simulink model "simplified_powertrain"  (R2020b)
settings: Solver=FixedStepAuto  StartTime=0.0  StopTime=60  RelTol=1e-3
PreLoadFcn:
  | C_sc = 1;
StartFcn:
  | C_sc = 1;
values from neighbouring files (symbols this model uses):
  D = 0    [model_fc.m]
undefined symbols (not defined in the file or in its folder): command, DiscIntNeverNeededParam, ECMS, Flight, in, Ion, Lithium, out, w
libraries: powerlib x22, electricdrivelib x3, lib_converters x3, simulink x2, fuzblock x1, mpclib x1, re_lib x1
(part 5 of 6)

== system simplified_powertrain/EMS/Management Variant/SMC/Discrete PI Controller1 ==
  note: Pierre Giroux, Gilbert Sybille
      | Power System Simulation Laboratory
      | IREQ, Hydro-Quebc
  note: Discrete PID Controller
  Error : Inport  SampleTime=Ts
  Discrete-Time Integrator : DiscreteIntegrator  InitialCondition=Init  SampleTime=Ts  LimitOutput=on  UpperSaturationLimit=UpperLimit  LowerSaturationLimit=LowerLimit  ICPrevOutput=DiscIntNeverNeededParam  ICPrevScaledInput=DiscIntNeverNeededParam
  Kp4 : Gain  Gain=Kp  SaturateOnIntegerOverflow=on  SampleTime=Ts  OutDataTypeStr=Inherit: Same as input  ParamDataTypeStr=Inherit: Same as input
  Kp5 : Gain  Gain=Ki  SaturateOnIntegerOverflow=on  SampleTime=Ts  OutDataTypeStr=Inherit: Same as input  ParamDataTypeStr=Inherit: Same as input
  Saturation2 : Saturate  UpperLimit=UpperLimit  LowerLimit=LowerLimit  SampleTime=Ts
  Sum6 : Sum  InputSameDT=on  SaturateOnIntegerOverflow=on  SampleTime=Ts  OutDataTypeStr=Inherit: Same as first input
  Zero-Order Hold : ZeroOrderHold  SampleTime=Ts
  Out : Outport  SampleTime=Ts  InitialOutput=0  VectorParamsAs1DForOutWhenUnconnected=off
  wires:
  Error/1 -> Kp4/1, Kp5/1
  Sum6/1 -> Saturation2/1
  Kp5/1 -> Discrete-Time Integrator/1
  Kp4/1 -> Zero-Order Hold/1
  Discrete-Time Integrator/1 -> Sum6/2
  Saturation2/1 -> Out/1
  Zero-Order Hold/1 -> Sum6/1

== system simplified_powertrain/EMS/Management Variant/SMC/Discrete PI Controller2 ==
  note: Pierre Giroux, Gilbert Sybille
      | Power System Simulation Laboratory
      | IREQ, Hydro-Quebc
  note: Discrete PID Controller
  Error : Inport  SampleTime=Ts
  Discrete-Time Integrator : DiscreteIntegrator  InitialCondition=Init  SampleTime=Ts  LimitOutput=on  UpperSaturationLimit=UpperLimit  LowerSaturationLimit=LowerLimit  ICPrevOutput=DiscIntNeverNeededParam  ICPrevScaledInput=DiscIntNeverNeededParam
  Kp4 : Gain  Gain=Kp  SaturateOnIntegerOverflow=on  SampleTime=Ts  OutDataTypeStr=Inherit: Same as input  ParamDataTypeStr=Inherit: Same as input
  Kp5 : Gain  Gain=Ki  SaturateOnIntegerOverflow=on  SampleTime=Ts  OutDataTypeStr=Inherit: Same as input  ParamDataTypeStr=Inherit: Same as input
  Saturation2 : Saturate  UpperLimit=UpperLimit  LowerLimit=LowerLimit  SampleTime=Ts
  Sum6 : Sum  InputSameDT=on  SaturateOnIntegerOverflow=on  SampleTime=Ts  OutDataTypeStr=Inherit: Same as first input
  Zero-Order Hold : ZeroOrderHold  SampleTime=Ts
  Out : Outport  SampleTime=Ts  InitialOutput=0  VectorParamsAs1DForOutWhenUnconnected=off
  wires:
  Error/1 -> Kp4/1, Kp5/1
  Sum6/1 -> Saturation2/1
  Kp5/1 -> Discrete-Time Integrator/1
  Kp4/1 -> Zero-Order Hold/1
  Discrete-Time Integrator/1 -> Sum6/2
  Saturation2/1 -> Out/1
  Zero-Order Hold/1 -> Sum6/1

== system simplified_powertrain/EMS/Management Variant/SMC/Discrete PI Controller3 ==
  note: Discrete PID Controller
  note: Pierre Giroux, Gilbert Sybille
      | Power System Simulation Laboratory
      | IREQ, Hydro-Quebc
  Error : Inport  SampleTime=Ts
  Discrete-Time Integrator : DiscreteIntegrator  InitialCondition=Init  SampleTime=Ts  LimitOutput=on  UpperSaturationLimit=UpperLimit  LowerSaturationLimit=LowerLimit  ICPrevOutput=DiscIntNeverNeededParam  ICPrevScaledInput=DiscIntNeverNeededParam
  Kp4 : Gain  Gain=Kp  SaturateOnIntegerOverflow=on  SampleTime=Ts  OutDataTypeStr=Inherit: Same as input  ParamDataTypeStr=Inherit: Same as input
  Kp5 : Gain  Gain=Ki  SaturateOnIntegerOverflow=on  SampleTime=Ts  OutDataTypeStr=Inherit: Same as input  ParamDataTypeStr=Inherit: Same as input
  Saturation2 : Saturate  UpperLimit=UpperLimit  LowerLimit=LowerLimit  SampleTime=Ts
  Sum6 : Sum  InputSameDT=on  SaturateOnIntegerOverflow=on  SampleTime=Ts  OutDataTypeStr=Inherit: Same as first input
  Zero-Order Hold : ZeroOrderHold  SampleTime=Ts
  Out : Outport  SampleTime=Ts  InitialOutput=0  VectorParamsAs1DForOutWhenUnconnected=off
  wires:
  Zero-Order Hold/1 -> Sum6/1
  Saturation2/1 -> Out/1
  Discrete-Time Integrator/1 -> Sum6/2
  Kp4/1 -> Zero-Order Hold/1
  Kp5/1 -> Discrete-Time Integrator/1
  Sum6/1 -> Saturation2/1
  Error/1 -> Kp5/1, Kp4/1

== system simplified_powertrain/EMS/Management Variant/SMC/Discrete PI Controller5 ==
  note: Pierre Giroux, Gilbert Sybille
      | Power System Simulation Laboratory
      | IREQ, Hydro-Quebc
  note: Discrete PID Controller
  Error : Inport  SampleTime=Ts
  Discrete-Time Integrator : DiscreteIntegrator  InitialCondition=Init  SampleTime=Ts  LimitOutput=on  UpperSaturationLimit=UpperLimit  LowerSaturationLimit=LowerLimit  ICPrevOutput=DiscIntNeverNeededParam  ICPrevScaledInput=DiscIntNeverNeededParam
  Kp4 : Gain  Gain=Kp  SaturateOnIntegerOverflow=on  SampleTime=Ts  OutDataTypeStr=Inherit: Same as input  ParamDataTypeStr=Inherit: Same as input
  Kp5 : Gain  Gain=Ki  SaturateOnIntegerOverflow=on  SampleTime=Ts  OutDataTypeStr=Inherit: Same as input  ParamDataTypeStr=Inherit: Same as input
  Saturation2 : Saturate  UpperLimit=UpperLimit  LowerLimit=LowerLimit  SampleTime=Ts
  Sum6 : Sum  InputSameDT=on  SaturateOnIntegerOverflow=on  SampleTime=Ts  OutDataTypeStr=Inherit: Same as first input
  Zero-Order Hold : ZeroOrderHold  SampleTime=Ts
  Out : Outport  SampleTime=Ts  InitialOutput=0  VectorParamsAs1DForOutWhenUnconnected=off
  wires:
  Error/1 -> Kp4/1, Kp5/1
  Sum6/1 -> Saturation2/1
  Kp5/1 -> Discrete-Time Integrator/1
  Kp4/1 -> Zero-Order Hold/1
  Discrete-Time Integrator/1 -> Sum6/2
  Saturation2/1 -> Out/1
  Zero-Order Hold/1 -> Sum6/1

== system simplified_powertrain/EMS/Management Variant/SMC/Discrete PI Controller6 ==
  note: Discrete PID Controller
  note: Pierre Giroux, Gilbert Sybille
      | Power System Simulation Laboratory
      | IREQ, Hydro-Quebc
  Error : Inport  SampleTime=Ts
  Discrete-Time Integrator : DiscreteIntegrator  InitialCondition=Init  SampleTime=Ts  LimitOutput=on  UpperSaturationLimit=UpperLimit  LowerSaturationLimit=LowerLimit  ICPrevOutput=DiscIntNeverNeededParam  ICPrevScaledInput=DiscIntNeverNeededParam
  Kp4 : Gain  Gain=Kp  SaturateOnIntegerOverflow=on  SampleTime=Ts  OutDataTypeStr=Inherit: Same as input  ParamDataTypeStr=Inherit: Same as input
  Kp5 : Gain  Gain=Ki  SaturateOnIntegerOverflow=on  SampleTime=Ts  OutDataTypeStr=Inherit: Same as input  ParamDataTypeStr=Inherit: Same as input
  Saturation2 : Saturate  UpperLimit=UpperLimit  LowerLimit=LowerLimit  SampleTime=Ts
  Sum6 : Sum  InputSameDT=on  SaturateOnIntegerOverflow=on  SampleTime=Ts  OutDataTypeStr=Inherit: Same as first input
  Zero-Order Hold : ZeroOrderHold  SampleTime=Ts
  Out : Outport  SampleTime=Ts  InitialOutput=0  VectorParamsAs1DForOutWhenUnconnected=off
  wires:
  Zero-Order Hold/1 -> Sum6/1
  Saturation2/1 -> Out/1
  Discrete-Time Integrator/1 -> Sum6/2
  Kp4/1 -> Zero-Order Hold/1
  Kp5/1 -> Discrete-Time Integrator/1
  Sum6/1 -> Saturation2/1
  Error/1 -> Kp5/1, Kp4/1

== system simplified_powertrain/EMS/Management Variant/SMC/Discrete PI Controller7 ==
  note: Pierre Giroux, Gilbert Sybille
      | Power System Simulation Laboratory
      | IREQ, Hydro-Quebc
  note: Discrete PID Controller
  Error : Inport  SampleTime=Ts
  Discrete-Time Integrator : DiscreteIntegrator  InitialCondition=Init  SampleTime=Ts  LimitOutput=on  UpperSaturationLimit=UpperLimit  LowerSaturationLimit=LowerLimit  ICPrevOutput=DiscIntNeverNeededParam  ICPrevScaledInput=DiscIntNeverNeededParam
  Kp4 : Gain  Gain=Kp  SaturateOnIntegerOverflow=on  SampleTime=Ts  OutDataTypeStr=Inherit: Same as input  ParamDataTypeStr=Inherit: Same as input
  Kp5 : Gain  Gain=Ki  SaturateOnIntegerOverflow=on  SampleTime=Ts  OutDataTypeStr=Inherit: Same as input  ParamDataTypeStr=Inherit: Same as input
  Saturation2 : Saturate  UpperLimit=UpperLimit  LowerLimit=LowerLimit  SampleTime=Ts
  Sum6 : Sum  InputSameDT=on  SaturateOnIntegerOverflow=on  SampleTime=Ts  OutDataTypeStr=Inherit: Same as first input
  Zero-Order Hold : ZeroOrderHold  SampleTime=Ts
  Out : Outport  SampleTime=Ts  InitialOutput=0  VectorParamsAs1DForOutWhenUnconnected=off
  wires:
  Error/1 -> Kp4/1, Kp5/1
  Sum6/1 -> Saturation2/1
  Kp5/1 -> Discrete-Time Integrator/1
  Kp4/1 -> Zero-Order Hold/1
  Discrete-Time Integrator/1 -> Sum6/2
  Saturation2/1 -> Out/1
  Zero-Order Hold/1 -> Sum6/1

== matlab function simplified_powertrain/EMS/Management Variant/SMC/MATLAB Function ==
  settings: updateMethod=DISCRETE  sampleTime=Ts
  data: Vbatt input; Ibatt input; Ibatt_out input; Ibatt_1 output; Ifc_out input; Vpv input; Ipv input; Ipv_out input; Pload input; Vdc input; Vdc_wanted input; Pout input; Ibatt_2 output; Ibatt_3 output; IO_batt_conv output; IO_batt_conv_value input; Ifc_boost input; Vfc input
function [Ibatt_1, Ibatt_2, Ibatt_3,  IO_batt_conv] = fcn(Vbatt, Ibatt,Ibatt_out, Ifc_out, Vpv, Ipv, Ipv_out,Pload,Vdc,Vdc_wanted, Pout, IO_batt_conv_value, Ifc_boost, Vfc)
    %% Part - 1
    %     FC = Vfc * Ifc_boost;
    %     FC = Vfc * Ifc_in;
    %     FC = Vdc_wanted * Ifc_out;
    FC = Vdc * Ifc_out;
    
    %     PV = Vpv * Ipv_boost;
%         PV = Vpv * Ipv; % stable pv panel but not good
    %     PV = Vdc_wanted * Ipv_out;
    PV = Vdc * Ipv_out; % marche mieux avec celui ci mais pv pas au max
    
    %     Batt = Vbatt * Ibatt;
    Batt = Vdc * Ibatt_out;
    
    %     Ibatt_1 = (Pload - FC - PV)/Vdc_wanted;
    %     Ibatt_1 = (Pload - FC - PV)/Vdc;
    Ibatt_1 = (Pload - FC - PV - Batt)/Vdc;
    %     Ibatt_1 = -10;
    
    %% Part - 2
    Ibatt_2 = Pload - Pout;
    
    %% Part - 3
    Ibatt_3 = Vdc_wanted - Vdc;
    
    %% Activate conv
    IO_batt_conv = IO_batt_conv_value;
end

== matlab function simplified_powertrain/MATLAB Function1 ==
  data: Pfc_in input; FC output; Pfc_out input; Pbatt_in input; Pbatt_out input; Ppv_in input; Ppv_out input; BATT output; PV output
function [FC,BATT,PV] = fcn(Pfc_in,Pfc_out,Pbatt_in,Pbatt_out,Ppv_in,Ppv_out)

    FC = 100*Pfc_out/Pfc_in;
    BATT = 100*Pbatt_out/Pbatt_in;
    PV = 100*Ppv_out/Ppv_in;
    
    if FC > 100
        FC = 100;
    end
    if FC< 0
        FC = 0;
    end
    if BATT > 100
        BATT = 100;
    end
    if BATT< 0
        BATT = 0;
    end
    if PV > 100
        PV = 100;
    end
    if PV< 0
        PV = 0;
    end
    
end

== matlab function simplified_powertrain/EMS/Management Variant/FUZZY/MATLAB Function ==
  settings: updateMethod=DISCRETE  sampleTime=Ts
  data: Vbatt input; Ibatt input; Ibatt_out input; Ibatt_1 output; Ifc_out input; Vpv input; Ipv input; Ipv_out input; Pload input; Vdc input; Vdc_wanted input; Pout input; Ibatt_2 output; Ibatt_3 output; IO_batt_conv output; IO_batt_conv_value input; Ifc_boost input; Vfc input
function [Ibatt_1, Ibatt_2, Ibatt_3,  IO_batt_conv] = fcn(Vbatt, Ibatt,Ibatt_out, Ifc_out, Vpv, Ipv, Ipv_out,Pload,Vdc,Vdc_wanted, Pout, IO_batt_conv_value, Ifc_boost, Vfc)
    %% Part - 1
    %     FC = Vfc * Ifc_boost;
    %     FC = Vfc * Ifc_in;
    %     FC = Vdc_wanted * Ifc_out;
    FC = Vdc * Ifc_out;
    
    %     PV = Vpv * Ipv_boost;
%         PV = Vpv * Ipv; % stable pv panel but not good
    %     PV = Vdc_wanted * Ipv_out;
    PV = Vdc * Ipv_out; % marche mieux avec celui ci mais pv pas au max
    
    %     Batt = Vbatt * Ibatt;
    Batt = Vdc * Ibatt_out;
    
    %     Ibatt_1 = (Pload - FC - PV)/Vdc_wanted;
    %     Ibatt_1 = (Pload - FC - PV)/Vdc;
    Ibatt_1 = (Pload - FC - PV - Batt)/Vdc;
    %     Ibatt_1 = -10;
    
    %% Part - 2
    Ibatt_2 = Pload - Pout;
    
    %% Part - 3
    Ibatt_3 = Vdc_wanted - Vdc;
    
    %% Activate conv
    IO_batt_conv = IO_batt_conv_value;
end

== matlab function simplified_powertrain/EMS/Management Variant/FUZZY/MATLAB Function1 ==
  settings: updateMethod=DISCRETE  sampleTime=Ts
  data: current_comm input; conv output; Pload input; Vbus_required input; current_command output; V_batt_conv output
function [conv, current_command,V_batt_conv] = fcn(current_comm, Pload, Vbus_required)
    if current_comm < 0
        conv = 1;
        V_batt_conv = Vbus_required; % (55)
%         V_batt_conv = 55; % (55)
    else
        conv = 0;
        V_batt_conv = Vbus_required;
    end
%     V_batt_conv = 120;
    current_command = current_comm;
end

%     if Pload == 0 || current_comm < 0
%         conv = 1;
%         V_batt_conv = 50;
%     else
%         conv = 0;
%         V_batt_conv = Vbus_required;
%     end
%     current_command = current_comm;

== matlab function simplified_powertrain/EMS/Management Variant/FUZZY/PV - FC - control ==
  settings: updateMethod=DISCRETE  sampleTime=Ts
  data: Time input; Vdc_command input; Vfc input; Ifc_in input; Vbatt input; Ibatt_in input; Vpv input; Ifc output; Vfc_conv output; IO_fc_conv output; Pload input; Ipv_in input; SOC input; Ipv output; Vpv_conv output; IO_pv_conv output; Ipvout input; Vdc_real input; Pout_real input; Control_pv output; IO_pv_conv_value input; IO_fc_conv_value input; Control_pv_choose_var input; fuzzy_out input
function [Ifc,Vfc_conv,IO_fc_conv,Ipv,Vpv_conv,IO_pv_conv,Control_pv] ...
        = fcn(Time, Vdc_command,Vfc,Ifc_in, Vbatt, Ibatt_in, Vpv, Pload,...
        Ipv_in, SOC, Ipvout, Vdc_real, Pout_real, IO_pv_conv_value,...
        IO_fc_conv_value, Control_pv_choose_var, fuzzy_out)
    
    
    %% PV - Test for pv panel algo in Cascade control
    persistent Ppv_pre Ppv_w_pre;
    dataType = 'double';
    
    if isempty(Ppv_pre)
        Ppv_pre=0;
        Ppv_w_pre = 200;
    end
    
    if Control_pv_choose_var == 0 % Auto
        Control_pv = 2; % 1 = MPPT | 2 = Cascade Control
    else
        Control_pv = Control_pv_choose_var;
    end
    
    % ?? utile pour le début mais ne fonctionne pas après
%         if Pload == 0 && Control_pv_choose_var == 0
%             Control_pv = 1;
%         end
    
    
    
    Ppv_out = Ipvout*Vdc_real;
    Ppv_in = Ipv_in*Vpv;
    Delta_PV = 0.5;
    Ppv_wanted = Ppv_in;
    
    if Control_pv == 2 % Cascade control
        if mod(Time,2e-4) == 0
            if Ppv_in < Ppv_pre
                Ppv_wanted  = Ppv_in - Delta_PV;
            end
            if Ppv_in > Ppv_pre
                Ppv_wanted  = Ppv_in + Delta_PV;
            end
        end
        if Ppv_out < 0
            Ppv_wanted = 180;
        end
        
        Ipv = Ppv_wanted/Vpv;
    else
        Ipv = 0;
    end
    Vpv_conv = Vdc_command;
    
    
    % PV converter operates ?
    IO_pv_conv = IO_pv_conv_value;
    
    Ppv_pre = Ppv_in;
    Ppv_w_pre = Ppv_wanted;
    
    
    
    %% Set current for the FC
    Ifc = fuzzy_out * 1100/Vfc;

    Vfc_conv = Vdc_command;
    if Ifc_in < Ifc
        Vfc_conv = 100;
    end
       
    
    % FC converter operates ?
    IO_fc_conv = IO_fc_conv_value;
    
end

== matlab function simplified_powertrain/EMS/Management Variant/PI/MATLAB Function ==
  settings: updateMethod=DISCRETE  sampleTime=Ts
  data: Vbatt input; Ibatt input; Ibatt_out input; Ibatt_1 output; Ifc_out input; Vpv input; Ipv input; Ipv_out input; Pload input; Vdc input; Vdc_wanted input; Pout input; Ibatt_2 output; Ibatt_3 output; IO_batt_conv output; IO_batt_conv_value input; Ifc_boost input; Vfc input
function [Ibatt_1, Ibatt_2, Ibatt_3,  IO_batt_conv] = fcn(Vbatt, Ibatt,Ibatt_out, Ifc_out, Vpv, Ipv, Ipv_out,Pload,Vdc,Vdc_wanted, Pout, IO_batt_conv_value, Ifc_boost, Vfc)
    %% Part - 1
    %     FC = Vfc * Ifc_boost;
    %     FC = Vfc * Ifc_in;
    %     FC = Vdc_wanted * Ifc_out;
    FC = Vdc * Ifc_out;
    
    %     PV = Vpv * Ipv_boost;
%         PV = Vpv * Ipv; % stable pv panel but not good
    %     PV = Vdc_wanted * Ipv_out;
    PV = Vdc * Ipv_out; % marche mieux avec celui ci mais pv pas au max
    
    %     Batt = Vbatt * Ibatt;
    Batt = Vdc * Ibatt_out;
    
    %     Ibatt_1 = (Pload - FC - PV)/Vdc_wanted;
    %     Ibatt_1 = (Pload - FC - PV)/Vdc;
    Ibatt_1 = (Pload - FC - PV - Batt)/Vdc;
    %     Ibatt_1 = -10;
    
    %% Part - 2
    Ibatt_2 = Pload - Pout;
    
    %% Part - 3
    Ibatt_3 = Vdc_wanted - Vdc;
    
    %% Activate conv
    IO_batt_conv = IO_batt_conv_value;
end

== matlab function simplified_powertrain/EMS/Management Variant/PI/MATLAB Function1 ==
  settings: updateMethod=DISCRETE  sampleTime=Ts
  data: current_comm input; conv output; Pload input; Vbus_required input; current_command output; V_batt_conv output
function [conv, current_command,V_batt_conv] = fcn(current_comm, Pload, Vbus_required)
    if current_comm < 0
        conv = 1;
        V_batt_conv = Vbus_required; % (55)
    else
        conv = 0;
        V_batt_conv = Vbus_required;
    end
%     V_batt_conv = 120;
    current_command = current_comm;
end

%     if Pload == 0 || current_comm < 0
%         conv = 1;
%         V_batt_conv = 50;
%     else
%         conv = 0;
%         V_batt_conv = Vbus_required;
%     end
%     current_command = current_comm;

== matlab function simplified_powertrain/EMS/Management Variant/PI/PV - FC - control ==
  settings: updateMethod=DISCRETE  sampleTime=Ts
  data: Time input; Vdc_command input; Vfc input; Ifc_in input; Vbatt input; Ibatt_in input; Vpv input; Ifc output; Vfc_conv output; IO_fc_conv output; Pload input; Ipv_in input; Ipv output; Vpv_conv output; IO_pv_conv output; Ipvout input; Vdc_real input; Pout_real input; Control_pv output; IO_pv_conv_value input; IO_fc_conv_value input; Control_pv_choose_var input; BATT_SOC input
function [Ifc,Vfc_conv,IO_fc_conv,Ipv,Vpv_conv,IO_pv_conv,Control_pv] = ...
        fcn(Time, Vdc_command,Vfc,Ifc_in, Vbatt, Ibatt_in, Vpv, Pload, ...
        Ipv_in, Ipvout, Vdc_real, Pout_real, IO_pv_conv_value, ...
        IO_fc_conv_value, Control_pv_choose_var, BATT_SOC)
    
    
    %% PV - MPPT P&O algo in Cascade control
    
    % Get previous values for the MPPT algo in Cascade control
    persistent Ppv_pre Ppv_w_pre;
    dataType = 'double';
    if isempty(Ppv_pre)
        Ppv_pre=0;
        Ppv_w_pre = 200;
    end
    
    
    % Set the control mode
    if Control_pv_choose_var == 0 % Auto
        Control_pv = 2; % 1 = MPPT | 2 = Cascade Control
    else
        Control_pv = Control_pv_choose_var;
    end
    
    % See if needed to implement (useful for the beginning but didn't work
    % for the next flight scheme)
    %         if Pload == 0 && Control_pv_choose_var == 0
    %             Control_pv = 1;
    %         end
    
    
    
    Ppv_out = Ipvout*Vdc_real;
    Ppv_in = Ipv_in*Vpv;
    Delta_PV = 0.5;
    Ppv_wanted = Ppv_in;
    
    if Control_pv == 2 % Cascade control
        if mod(Time,2e-4) == 0
            if Ppv_in < Ppv_pre
                Ppv_wanted  = Ppv_in - Delta_PV;
            end
            if Ppv_in > Ppv_pre
                Ppv_wanted  = Ppv_in + Delta_PV;
            end
        end
        if Ppv_out < 0
            Ppv_wanted = 180;
        end
        
        Ipv = Ppv_wanted/Vpv;
    else
        Ipv = 0;
    end
    
    % Converter wanted output voltage
    Vpv_conv = Vdc_command;
    
    
    % PV converter operates ?
    IO_pv_conv = IO_pv_conv_value;
    
    
    % Set the values for the next loop
    Ppv_pre = Ppv_in;
    Ppv_w_pre = Ppv_wanted;
    
    
    
    
    %% FC - control
    % Set the error value for the PI
    Ifc = 50 - BATT_SOC;
    
    % Converter wanted output voltage
    Vfc_conv = Vdc_command;
    if BATT_SOC < 50
        Vfc_conv = 100;
    end
    
    % FC converter operates ?
    IO_fc_conv = IO_fc_conv_value;
    
end

== matlab function simplified_powertrain/EMS/Management Variant/ECMS/MATLAB Function ==
  settings: updateMethod=DISCRETE  sampleTime=Ts
  data: Vbatt input; Ibatt input; Ibatt_out input; Ibatt_1 output; Ifc_out input; Vpv input; Ipv input; Ipv_out input; Pload input; Vdc input; Vdc_wanted input; Pout input; Ibatt_2 output; Ibatt_3 output; IO_batt_conv output; IO_batt_conv_value input; Ifc_boost input; Vfc input
function [Ibatt_1, Ibatt_2, Ibatt_3,  IO_batt_conv] = fcn(Vbatt, Ibatt,Ibatt_out, Ifc_out, Vpv, Ipv, Ipv_out,Pload,Vdc,Vdc_wanted, Pout, IO_batt_conv_value, Ifc_boost, Vfc)
    %% Part - 1
    %     FC = Vfc * Ifc_boost;
    %     FC = Vfc * Ifc_in;
    %     FC = Vdc_wanted * Ifc_out;
    FC = Vdc * Ifc_out;
    
    %     PV = Vpv * Ipv_boost;
%         PV = Vpv * Ipv; % stable pv panel but not good
    %     PV = Vdc_wanted * Ipv_out;
    PV = Vdc * Ipv_out; % marche mieux avec celui ci mais pv pas au max
    
    %     Batt = Vbatt * Ibatt;
    Batt = Vdc * Ibatt_out;
    
    %     Ibatt_1 = (Pload - FC - PV)/Vdc_wanted;
    %     Ibatt_1 = (Pload - FC - PV)/Vdc;
    Ibatt_1 = (Pload - FC - PV - Batt)/Vdc;
    %     Ibatt_1 = -10;
    
    %% Part - 2
    Ibatt_2 = Pload - Pout;
    
    %% Part - 3
    Ibatt_3 = Vdc_wanted - Vdc;
    
    %% Activate conv
    IO_batt_conv = IO_batt_conv_value;
end

== matlab function simplified_powertrain/EMS/Management Variant/ECMS/MATLAB Function1 ==
  settings: updateMethod=DISCRETE  sampleTime=Ts
  data: current_comm input; conv output; Pload input; Vbus_required input; current_command output; V_batt_conv output
function [conv, current_command,V_batt_conv] = fcn(current_comm, Pload, Vbus_required)
    if current_comm < 0
        conv = 1;
        V_batt_conv = Vbus_required; % (55)
    else
        conv = 0;
        V_batt_conv = Vbus_required;
    end
%     V_batt_conv = 120;
    current_command = current_comm;
end

%     if Pload == 0 || current_comm < 0
%         conv = 1;
%         V_batt_conv = 50;
%     else
%         conv = 0;
%         V_batt_conv = Vbus_required;
%     end
%     current_command = current_comm;

== matlab function simplified_powertrain/EMS/Management Variant/ECMS/PV - FC - control ==
  settings: updateMethod=DISCRETE  sampleTime=Ts
  data: Time input; Vdc_command input; Vfc input; Ifc_in input; Vbatt input; Ibatt_in input; Vpv input; Ifc output; Vfc_conv output; IO_fc_conv output; Pload input; Ipv_in input; SOC input; Ipv output; Vpv_conv output; IO_pv_conv output; Ipvout input; Vdc_real input; Pout_real input; Control_pv output; IO_pv_conv_value input; IO_fc_conv_value input; Control_pv_choose_var input; BATT_SOC input
function [Ifc,Vfc_conv,IO_fc_conv,Ipv,Vpv_conv,IO_pv_conv,Control_pv] = ...
        fcn(Time, Vdc_command,Vfc,Ifc_in, Vbatt, Ibatt_in, Vpv, Pload, ...
        Ipv_in, SOC, Ipvout, Vdc_real, Pout_real, IO_pv_conv_value, ...
        IO_fc_conv_value, Control_pv_choose_var, BATT_SOC)
    
    
    %% PV - MPPT P&O algo in Cascade control
    % Get previous values for the MPPT algo in Cascade control
    persistent Ppv_pre Ppv_w_pre;
    dataType = 'double';
    if isempty(Ppv_pre)
        Ppv_pre=0;
        Ppv_w_pre = 200;
    end
    
    
    % Set the control mode
    if Control_pv_choose_var == 0 % Auto
        Control_pv = 2; % 1 = MPPT | 2 = Cascade Control
    else
        Control_pv = Control_pv_choose_var;
    end
        
    
    Ppv_out = Ipvout*Vdc_real;
    Ppv_in = Ipv_in*Vpv;
    Delta_PV = 0.5;
    Ppv_wanted = Ppv_in;
    
    if Control_pv == 2 % Cascade control
        if mod(Time,2e-4) == 0
            if Ppv_in < Ppv_pre
                Ppv_wanted  = Ppv_in - Delta_PV;
            end
            if Ppv_in > Ppv_pre
                Ppv_wanted  = Ppv_in + Delta_PV;
            end
        end
        if Ppv_out < 0
            Ppv_wanted = 180;
        end
        
        Ipv = Ppv_wanted/Vpv;
    else
        Ipv = 0;
    end
    
    % Converter wanter output voltage
    Vpv_conv = Vdc_command;
    
    
    % PV converter operates ?
    IO_pv_conv = IO_pv_conv_value;
    
    
    % Set the values for the next loop
    Ppv_pre = Ppv_in;
    Ppv_w_pre = Ppv_wanted;
    
    
    
    
    %% FC - control
    % FC converter operates ?
    IO_fc_conv = IO_fc_conv_value;
    
    % ECMS:
    Pbatt_min=-150; Pbatt_max=800;
    SOC_min=60; SOC_max=90; 
    Pfc_min=400;Pfc_max=1100; 

    %define Matrix Aeq

    Aeq=[0 1 0;1 0 1];

    %define Matrix beq
    mu=0.6;
    beq=[1-2*mu*((SOC-0.5*(SOC_max+SOC_min))/(SOC_max+SOC_min)); Pload-Ppv_out];

    %define boundary conditions
    lb=[Pfc_min, 0, Pbatt_min];
    ub=[Pfc_max, 100, Pbatt_max];

    %define initial conditions
    x0=[1000, 0.1, 500];
    options = optimoptions('fmincon','Algorithm','sqp',...
        'Display','off','MaxFunctionEvaluations',500,'MaxIterations',100);
    [y,fval] = fmincon(@ecms,x0,[],[],Aeq,beq,lb,ub,[],options);

    Pfc=y(1); Pbatt=y(3); alpha=y(2);
    Ifc = Pfc/Vfc;
    
    % Converter wanted output voltage
    Vfc_conv = Vdc_command;
    if Ifc_in < Ifc
        Vfc_conv = 100;
    end
    
function f = ecms(x)
DT=200e-3;
f = (x(1)+x(2)*x(3))*DT;

== matlab function simplified_powertrain/EMS/Management Variant/EEMS/MATLAB Function ==
  settings: updateMethod=DISCRETE  sampleTime=Ts
  data: Vbatt input; Ibatt input; Ibatt_out input; Ibatt_1 output; Ifc_out input; Vpv input; Ipv input; Ipv_out input; Pload input; Vdc input; Vdc_wanted input; Pout input; Ibatt_2 output; Ibatt_3 output; IO_batt_conv output; IO_batt_conv_value input; Ifc_boost input; Vfc input
function [Ibatt_1, Ibatt_2, Ibatt_3,  IO_batt_conv] = fcn(Vbatt, Ibatt,Ibatt_out, Ifc_out, Vpv, Ipv, Ipv_out,Pload,Vdc,Vdc_wanted, Pout, IO_batt_conv_value, Ifc_boost, Vfc)
    %% Part - 1
    %     FC = Vfc * Ifc_boost;
    %     FC = Vfc * Ifc_in;
    %     FC = Vdc_wanted * Ifc_out;
    FC = Vdc * Ifc_out;
    
    %     PV = Vpv * Ipv_boost;
%         PV = Vpv * Ipv; % stable pv panel but not good
    %     PV = Vdc_wanted * Ipv_out;
    PV = Vdc * Ipv_out; % marche mieux avec celui ci mais pv pas au max
    
    %     Batt = Vbatt * Ibatt;
    Batt = Vdc * Ibatt_out;
    
    %     Ibatt_1 = (Pload - FC - PV)/Vdc_wanted;
    %     Ibatt_1 = (Pload - FC - PV)/Vdc;
    Ibatt_1 = (Pload - FC - PV - Batt)/Vdc;
    %     Ibatt_1 = -10;
    
    %% Part - 2
    Ibatt_2 = Pload - Pout;
    
    %% Part - 3
    Ibatt_3 = Vdc_wanted - Vdc;
    
    %% Activate conv
    IO_batt_conv = IO_batt_conv_value;
end

== matlab function simplified_powertrain/EMS/Management Variant/EEMS/MATLAB Function1 ==
  settings: updateMethod=DISCRETE  sampleTime=Ts
  data: current_comm input; conv output; Pload input; Vbus_required input; current_command output; V_batt_conv output; DV input
function [conv, current_command,V_batt_conv] = fcn(current_comm, Pload, Vbus_required, DV)
    if current_comm < 0
        conv = 1;
        V_batt_conv = Vbus_required; % (55)
    else
        conv = 0;
        V_batt_conv = Vbus_required;
    end
%     V_batt_conv = 120;
    current_command = current_comm;
    Vbatt_conv = V_batt_conv + DV;
end

%     if Pload == 0 || current_comm < 0
%         conv = 1;
%         V_batt_conv = 50;
%     else
%         conv = 0;
%         V_batt_conv = Vbus_required;
%     end
%     current_command = current_comm;

== matlab function simplified_powertrain/EMS/Management Variant/SMC/PV - FC - control ==
  settings: updateMethod=DISCRETE  sampleTime=Ts
  data: Time input; Vdc_command input; Vfc input; Ifc_in input; Vbatt input; Ibatt_in input; Vpv input; Ifc output; Vfc_conv output; IO_fc_conv output; Pload input; Ipv_in input; Ipv output; Vpv_conv output; IO_pv_conv output; Ipvout input; Vdc_real input; Pout_real input; Control_pv output; IO_pv_conv_value input; IO_fc_conv_value input; Control_pv_choose_var input; BATT_SOC input
function [Ifc,Vfc_conv,IO_fc_conv,Ipv,Vpv_conv,IO_pv_conv,Control_pv] = ...
        fcn(Time, Vdc_command,Vfc,Ifc_in, Vbatt, Ibatt_in, Vpv, Pload, ...
        Ipv_in, Ipvout, Vdc_real, Pout_real, IO_pv_conv_value, ...
        IO_fc_conv_value, Control_pv_choose_var,BATT_SOC)
    
    
    %% PV - MPPT P&O algo in Cascade control
    % Get previous values for the MPPT algo in Cascade control
    persistent Ppv_pre Ppv_w_pre;
    dataType = 'double';
    if isempty(Ppv_pre)
        Ppv_pre=0;
        Ppv_w_pre = 200;
    end
    
    
    % Set the control mode
    if Control_pv_choose_var == 0 % Auto
        Control_pv = 2; % 1 = MPPT | 2 = Cascade Control
    else
        Control_pv = Control_pv_choose_var;
    end
    
    % See if needed to implement (useful for the beginning but didn't work
    % for the next flight scheme)
    %         if Pload == 0 && Control_pv_choose_var == 0
    %             Control_pv = 1;
    %         end
    
    
    
    Ppv_out = Ipvout*Vdc_real;
    Ppv_in = Ipv_in*Vpv;
    Delta_PV = 0.5;
    Ppv_wanted = Ppv_in;
    
    if Control_pv == 2 % Cascade control
        if mod(Time,2e-4) == 0
            if Ppv_in < Ppv_pre
                Ppv_wanted  = Ppv_in - Delta_PV;
            end
            if Ppv_in > Ppv_pre
                Ppv_wanted  = Ppv_in + Delta_PV;
            end
        end
        if Ppv_out < 0
            Ppv_wanted = 180;
        end
        
        Ipv = Ppv_wanted/Vpv;
    else
        Ipv = 0;
    end
    
    % Converter wanted output voltage
    Vpv_conv = Vdc_command;
    
    
    % PV converter operates ?
    IO_pv_conv = IO_pv_conv_value;
    
    
    % Set the values for the next loop
    Ppv_pre = Ppv_in;
    Ppv_w_pre = Ppv_wanted;
    
    
    
    
    %% FC - control
    % Set / get previous data
    persistent pre_condition;
    if isempty(pre_condition)
        pre_condition=0;
    end
    
    
    % Set boundaries
    % batt
    SOC_min = 35;
    SOC_lb = 45;
    SOC_ub = 75;
    SOC_max = 85;
    
    % fuel cell
    Pfc_min = 500;
    Pfc_rated = 1000;
    Pfc_max = 1100;
    Pfc_command = Pfc_rated;
    
    % Change Pout by Pload - Ppv_out ? % risk of bug ?
%     Pout = Pload;
    Pout = Pload - Ppv_out;
    
    %%  Condition + command
    cur_condition = 1;
    if BATT_SOC < SOC_min
        cur_condition = 1;
    end
    if BATT_SOC >= SOC_min && BATT_SOC < SOC_lb
        cur_condition = pre_condition;
    end
    if BATT_SOC >= SOC_lb && BATT_SOC <= SOC_ub
        cur_condition = 2;
    end
    if BATT_SOC >= SOC_ub && BATT_SOC < SOC_max
        cur_condition = pre_condition;
    end
    if BATT_SOC > SOC_max
        cur_condition = 3;
    end
    
    
    if cur_condition == 1 && Pout < Pfc_min
        Pfc_command = Pfc_max; % need to change (get value of the max / typical
        % power to charge the battery)
    end
    if cur_condition == 1 && Pout >= Pfc_min && Pout <= Pfc_rated
        Pfc_command = Pfc_rated; % need to change (get value of the max / typical
        % power to charge the battery)
    end
    if cur_condition == 1 && Pout >= Pfc_rated && Pout <= Pfc_max
        Pfc_command = Pfc_max; % need to change (get value of the max / typical
        % power to charge the battery)
    end
    if cur_condition == 1 && Pout > Pfc_max
        Pfc_command = Pfc_max;
    end
    
    if cur_condition == 2 && Pout < Pfc_min
        Pfc_command = Pfc_min;
    end
    if cur_condition == 2 && Pout >= Pfc_min && Pout <= Pfc_rated
        Pfc_command = Pfc_rated;
    end
    if cur_condition == 2 && Pout >= Pfc_rated && Pout <= Pfc_max
        Pfc_command = Pout;
    end
    if cur_condition == 2 && Pout > Pfc_max
        Pfc_command = Pfc_rated;
    end
    
    if cur_condition == 3 && Pout < Pfc_min
        Pfc_command = Pfc_min;
    end
    if cur_condition == 3 && Pout >= Pfc_min && Pout <= Pfc_rated
        Pfc_command = Pout;
    end
    

    %% Set output
    % set the pre_condition value:
    pre_condition = cur_condition;
    
    % Converter current command
    Ifc = Pfc_command / Vfc;
    
    % Converter wanted output voltage
    Vfc_conv = Vdc_command;
    if Ifc_in < Ifc
        Vfc_conv = 100;
    end % doesn't work as expected
    
    
    % FC converter operates ?
    IO_fc_conv = IO_fc_conv_value;
    
end

== matlab function simplified_powertrain/EMS/Management Variant/EEMS/PV - FC - control ==
  settings: updateMethod=DISCRETE  sampleTime=Ts
  data: Time input; Vdc_command input; Vfc input; Ifc_in input; Vbatt input; Ibatt_in input; Vpv input; Ifc output; Vfc_conv output; IO_fc_conv output; Pload input; Ipv_in input; SOC input; Ipv output; Vpv_conv output; IO_pv_conv output; Ipvout input; Vdc_real input; Pout_real input; Control_pv output; IO_pv_conv_value input; IO_fc_conv_value input; Control_pv_choose_var input; BATT_SOC input; DV output
function [Ifc,Vfc_conv,IO_fc_conv,Ipv,Vpv_conv,IO_pv_conv,Control_pv,DV] = ...
        fcn(Time, Vdc_command,Vfc,Ifc_in, Vbatt, Ibatt_in, Vpv, Pload, ...
        Ipv_in, SOC, Ipvout, Vdc_real, Pout_real, IO_pv_conv_value, ...
        IO_fc_conv_value, Control_pv_choose_var, BATT_SOC)
    
    
    %% PV - MPPT P&O algo in Cascade control
    % Get previous values for the MPPT algo in Cascade control
    persistent Ppv_pre Ppv_w_pre;
    dataType = 'double';
    if isempty(Ppv_pre)
        Ppv_pre=0;
        Ppv_w_pre = 200;
    end
    
    
    % Set the control mode
    if Control_pv_choose_var == 0 % Auto
        Control_pv = 2; % 1 = MPPT | 2 = Cascade Control
    else
        Control_pv = Control_pv_choose_var;
    end
    
    % See if needed to implement (useful for the beginning but didn't work
    % for the next flight scheme)
    %         if Pload == 0 && Control_pv_choose_var == 0
    %             Control_pv = 1;
    %         end
    
    
    
    Ppv_out = Ipvout*Vdc_real;
    Ppv_in = Ipv_in*Vpv;
    Delta_PV = 0.5;
    Ppv_wanted = Ppv_in;
    
    if Control_pv == 2 % Cascade control
        if mod(Time,2e-4) == 0
            if Ppv_in < Ppv_pre
                Ppv_wanted  = Ppv_in - Delta_PV;
            end
            if Ppv_in > Ppv_pre
                Ppv_wanted  = Ppv_in + Delta_PV;
            end
        end
        if Ppv_out < 0
            Ppv_wanted = 180;
        end
        
        Ipv = Ppv_wanted/Vpv;
    else
        Ipv = 0;
    end
    
    % Converter wanter output voltage
    Vpv_conv = Vdc_command;
    
    
    % PV converter operates ?
    IO_pv_conv = IO_pv_conv_value;
    
    
    % Set the values for the next loop
    Ppv_pre = Ppv_in;
    Ppv_w_pre = Ppv_wanted;
    
    
    
    
    %% FC - control    
    % Converter wanter output voltage
    Vfc_conv = Vdc_command;
    if BATT_SOC < 50
        Vfc_conv = 100;
    end
    
    % FC converter operates ?
    IO_fc_conv = IO_fc_conv_value;
    
    %% EEMS
    %constants initialization
    Pbatt_min=-150; Pbatt_max=800;
    SOC_min=60; Q=36*15;
    DV_min=-0.5; DV_max=0.5;
    DT=200e-3; 
    Vbatt_nom=48;
    Vdc_min=71.5;
    % define matrix A
    
    A = [DT 0;0 -1];
    
    %define matrix b
    
    b =[(SOC-SOC_min)*Vbatt_nom*Q; Vdc_real-Vdc_min];
    %define boundary conditions
    lb=[Pbatt_min, DV_min];
    ub=[Pbatt_max, DV_max];
    %define initial conditions
    x0=[Pbatt_max, DV_min];
    options = optimoptions('fmincon','Algorithm','sqp','Display','off','MaxFunctionEvaluations',500,'MaxIterations',100);
    [y,fval] = fmincon(@eemsfun,x0,A,b,[],[],lb,ub,[],options); %#ok<*ASGLU>
    Pbatt=y(1); DV=y(2);
    
    Ifc = (Pload - Pbatt)/Vfc;
    
function f = eemsfun(x)
    DT=200e-3;
    C=1;
    f = -x(1)*DT- 0.5*C*x(2)^2;

== matlab function simplified_powertrain/EMS/Management Variant/Constant/MATLAB Function ==
  settings: updateMethod=DISCRETE  sampleTime=Ts
  data: Vbatt input; Ibatt input; Ibatt_out input; Ibatt_1 output; Ifc_out input; Vpv input; Ipv input; Ipv_out input; Pload input; Vdc input; Vdc_wanted input; Pout input; Ibatt_2 output; Ibatt_3 output; IO_batt_conv output; IO_batt_conv_value input; Ifc_boost input; Vfc input
function [Ibatt_1, Ibatt_2, Ibatt_3,  IO_batt_conv] = fcn(Vbatt, Ibatt,Ibatt_out, Ifc_out, Vpv, Ipv, Ipv_out,Pload,Vdc,Vdc_wanted, Pout, IO_batt_conv_value, Ifc_boost, Vfc)
    %% Part - 1
    %     FC = Vfc * Ifc_boost;
    %     FC = Vfc * Ifc_in;
    %     FC = Vdc_wanted * Ifc_out;
    FC = Vdc * Ifc_out;
    
    %     PV = Vpv * Ipv_boost;
%         PV = Vpv * Ipv; % stable pv panel but not good
    %     PV = Vdc_wanted * Ipv_out;
    PV = Vdc * Ipv_out; % marche mieux avec celui ci mais pv pas au max
    
    %     Batt = Vbatt * Ibatt;
    Batt = Vdc * Ibatt_out;
    
    %     Ibatt_1 = (Pload - FC - PV)/Vdc_wanted;
    %     Ibatt_1 = (Pload - FC - PV)/Vdc;
    Ibatt_1 = (Pload - FC - PV - Batt)/Vdc;
    %     Ibatt_1 = -10;
    
    %% Part - 2
    Ibatt_2 = Pload - Pout;
    
    %% Part - 3
    Ibatt_3 = Vdc_wanted - Vdc;
    
    %% Activate conv
    IO_batt_conv = IO_batt_conv_value;
end

== matlab function simplified_powertrain/EMS/Management Variant/Constant/MATLAB Function1 ==
  settings: updateMethod=DISCRETE  sampleTime=Ts
  data: current_comm input; conv output; Pload input; Vbus_required input; current_command output; V_batt_conv output
function [conv, current_command,V_batt_conv] = fcn(current_comm, Pload, Vbus_required)
    if current_comm < 0
        conv = 1;
        V_batt_conv = Vbus_required; % (55)
    else
        conv = 0;
        V_batt_conv = Vbus_required;
    end
%     V_batt_conv = 120;
    current_command = current_comm;
end

%     if Pload == 0 || current_comm < 0
%         conv = 1;
%         V_batt_conv = 50;
%     else
%         conv = 0;
%         V_batt_conv = Vbus_required;
%     end
%     current_command = current_comm;

== matlab function simplified_powertrain/EMS/Management Variant/Constant/PV - FC - control ==
  settings: updateMethod=DISCRETE  sampleTime=Ts
  data: Time input; Vdc_command input; Vfc input; Ifc_in input; Vbatt input; Ibatt_in input; Vpv input; Ifc output; Vfc_conv output; IO_fc_conv output; Pload input; Ipv_in input; SOC input; Ipv output; Vpv_conv output; IO_pv_conv output; Ipvout input; Vdc_real input; Pout_real input; Control_pv output; IO_pv_conv_value input; IO_fc_conv_value input; Control_pv_choose_var input
function [Ifc,Vfc_conv,IO_fc_conv,Ipv,Vpv_conv,IO_pv_conv,Control_pv] = fcn(Time, Vdc_command,Vfc,Ifc_in, Vbatt, Ibatt_in, Vpv, Pload, Ipv_in, SOC, Ipvout, Vdc_real, Pout_real, IO_pv_conv_value, IO_fc_conv_value, Control_pv_choose_var)
    
    
    %% Test for pv panel P&O algo
    persistent Ppv_pre Ppv_w_pre;
    dataType = 'double';
    
    if isempty(Ppv_pre)
        Ppv_pre=0;
        Ppv_w_pre = 200;
    end
    
    if Control_pv_choose_var == 0 % Auto
        Control_pv = 2; % 1 = MPPT | 2 = Cascade Control
    else
        Control_pv = Control_pv_choose_var;
    end
    
    % ?? utile pour le début mais ne fonctionne pas après
%         if Pload == 0 && Control_pv_choose_var == 0
%             Control_pv = 1;
%         end
    
    
    
    Ppv_out = Ipvout*Vdc_real;
    Ppv_in = Ipv_in*Vpv;
    Delta_PV = 0.5;
    Ppv_wanted = Ppv_in;
    
    if Control_pv == 2 % Cascade control
        if mod(Time,2e-4) == 0
            if Ppv_in < Ppv_pre
                Ppv_wanted  = Ppv_in - Delta_PV;
            end
            if Ppv_in > Ppv_pre
                Ppv_wanted  = Ppv_in + Delta_PV;
            end
        end
        if Ppv_out < 0
            Ppv_wanted = 180;
        end
        
        Ipv = Ppv_wanted/Vpv;
    else
        Ipv = 0;
    end
%         Ipv = 180/Vpv;
    Vpv_conv = Vdc_command;
    
    
    % PV converter operates ?
    IO_pv_conv = IO_pv_conv_value;
    
    Ppv_pre = Ppv_in;
    Ppv_w_pre = Ppv_wanted;
    
    
    %% Set if needed
    %     Ipv = 185/Vpv;
    
    
    %% Set max current wanted for the fuel cell
    %     Ifc = 200/Vfc; % doesn't work with my own model
    %     Ifc = 7; % doesn't work with battery ??
    Ifc = 1100/Vfc; % work now ??

    Vfc_conv = Vdc_command;
    if Ifc_in < Ifc
        Vfc_conv = 100;
    end

    
    % FC converter operates ?
    IO_fc_conv = IO_fc_conv_value;
    
end

== matlab function simplified_powertrain/PV MODULE1/PV_function ==
  settings: updateMethod=DISCRETE  sampleTime=Ts
  data: TempCell_C input; ID output; Irradiance input; Ncell input; Voc input; Isc input; Vmp input; Imp input; alpha input; beta input; IPH_STC input; I_0 input; V_PV input; I_PV input; a input; Rp input; Rs input; para_string input; serie_string input
function ID = pv_calculation(TempCell_C, Irradiance, Ncell, Voc, Isc, Vmp, Imp, alpha, beta, IPH_STC, I_0,V_PV, I_PV, a, Rp, Rs, para_string, serie_string)
    %% Constant
    n = a;
    Tc_STC = 25 + 273.15;
    G_STC = 1000;
    TempCell_K = TempCell_C+273.15;
    
    k = 1.3806e-23; % Boltzman constant (J/K)
    k_ = 8.617333262145e-5; % Boltzman constant (eV/K)
    q = 1.602e-19; % Elementary charge on an electron (C)
    % k_ = k/q;
    Eg0 = 1.121;
    Eg_ref = Eg0*q; % Band gap for silicon (eV)
    
    
    

%     
%     if isnan(V_PV)
%         V_PV = 0;
%     end
%     if isnan(I_PV)
%         I_PV = 0;
%     end
    
    
    %% Method 2 + Ncell dans Id + -1 dans Irs + Ish différent
    %     Voc = Voc / Ncell;
    k = 1.3806e-23;
    Vt = k/q*TempCell_K;
    IPH = ((TempCell_K-Tc_STC)*alpha+IPH_STC)*para_string*Irradiance/G_STC;
    Ish = (V_PV + I_PV*Rs)/Rp;
    Irs = IPH_STC/(exp(q*Voc/(Ncell*k*a*TempCell_K))-1);
    Is = Irs * (TempCell_K/Tc_STC)^3*exp((Eg_ref/(k_*a))*(1/TempCell_K - 1/Tc_STC));
    % Maybe change above ? (1/Tc_STC - 1/TempCell_K) ??
    Id = para_string * Is * (exp((V_PV/serie_string+I_PV*Rs/para_string)/(n*Vt*Ncell))-1);
    ID = IPH * para_string - Ish - Id;
    
end


% https://hal.archives-ouvertes.fr/hal-01351308/document
% PV -> autre -> Matlab sim model
% PV -> autre -> PV panel
% PV -> autre -> PV module
% https://environmentalsystemsresearch.springeropen.com/articles/10.1186/s40068-015-0047-9
% https://iopscience.iop.org/article/10.1088/1757-899X/114/1/012137/pdf

== matlab function simplified_powertrain/EMS/Management Variant/D-ECMS/MATLAB Function ==
  settings: updateMethod=DISCRETE  sampleTime=Ts
  data: Vbatt input; Ibatt input; Ibatt_out input; Ibatt_1 output; Ifc_out input; Vpv input; Ipv input; Ipv_out input; Pload input; Vdc input; Vdc_wanted input; Pout input; Ibatt_2 output; Ibatt_3 output; IO_batt_conv output; IO_batt_conv_value input; Ifc_boost input; Vfc input
function [Ibatt_1, Ibatt_2, Ibatt_3,  IO_batt_conv] = fcn(Vbatt, Ibatt,Ibatt_out, Ifc_out, Vpv, Ipv, Ipv_out,Pload,Vdc,Vdc_wanted, Pout, IO_batt_conv_value, Ifc_boost, Vfc)
    %% Part - 1
    %     FC = Vfc * Ifc_boost;
    %     FC = Vfc * Ifc_in;
    %     FC = Vdc_wanted * Ifc_out;
    FC = Vdc * Ifc_out;
    
    %     PV = Vpv * Ipv_boost;
%         PV = Vpv * Ipv; % stable pv panel but not good
    %     PV = Vdc_wanted * Ipv_out;
    PV = Vdc * Ipv_out; % marche mieux avec celui ci mais pv pas au max
    
    %     Batt = Vbatt * Ibatt;
    Batt = Vdc * Ibatt_out;
    
    %     Ibatt_1 = (Pload - FC - PV)/Vdc_wanted;
    %     Ibatt_1 = (Pload - FC - PV)/Vdc;
    Ibatt_1 = (Pload - FC - PV - Batt)/Vdc;
    %     Ibatt_1 = -10;
    
    %% Part - 2
    Ibatt_2 = Pload - Pout;
    
    %% Part - 3
    Ibatt_3 = Vdc_wanted - Vdc;
    
    %% Activate conv
    IO_batt_conv = IO_batt_conv_value;
end

== matlab function simplified_powertrain/EMS/Management Variant/D-ECMS/MATLAB Function1 ==
  settings: updateMethod=DISCRETE  sampleTime=Ts
  data: current_comm input; conv output; Pload input; Vbus_required input; current_command output; V_batt_conv output
function [conv, current_command,V_batt_conv] = fcn(current_comm, Pload, Vbus_required)
    if current_comm < 0
        conv = 1;
        V_batt_conv = Vbus_required; % (55)
    else
        conv = 0;
        V_batt_conv = Vbus_required;
    end
%     V_batt_conv = 120;
    current_command = current_comm;
end

%     if Pload == 0 || current_comm < 0
%         conv = 1;
%         V_batt_conv = 50;
%     else
%         conv = 0;
%         V_batt_conv = Vbus_required;
%     end
%     current_command = current_comm;

== matlab function simplified_powertrain/EMS/Management Variant/D-ECMS/PV - FC - control ==
  settings: updateMethod=DISCRETE  sampleTime=Ts
  data: Time input; Vdc_command input; Vfc input; Ifc_in input; Vbatt input; Ibatt_in input; Vpv input; Ifc output; Vfc_conv output; IO_fc_conv output; Pload input; Ipv_in input; SOC input; Ipv output; Vpv_conv output; IO_pv_conv output; Ipvout input; Vdc_real input; Pout_real input; Control_pv output; IO_pv_conv_value input; IO_fc_conv_value input; Control_pv_choose_var input; BATT_SOC input
function [Ifc,Vfc_conv,IO_fc_conv,Ipv,Vpv_conv,IO_pv_conv,Control_pv] = ...
        fcn(Time, Vdc_command,Vfc,Ifc_in, Vbatt, Ibatt_in, Vpv, Pload, ...
        Ipv_in, SOC, Ipvout, Vdc_real, Pout_real, IO_pv_conv_value, ...
        IO_fc_conv_value, Control_pv_choose_var, BATT_SOC)
    
%     Degradation-Conscious Equivalent Consumption Minimization Strategy for a Fuel Cell Hybrid System
    %% PV - MPPT P&O algo in Cascade control
    % Get previous values for the MPPT algo in Cascade control
    persistent Ppv_pre Ppv_w_pre;
    dataType = 'double';
    if isempty(Ppv_pre)
        Ppv_pre=0;
        Ppv_w_pre = 200;
    end
    
    
    % Set the control mode
    if Control_pv_choose_var == 0 % Auto
        Control_pv = 2; % 1 = MPPT | 2 = Cascade Control
    else
        Control_pv = Control_pv_choose_var;
    end
    
    
    Ppv_out = Ipvout*Vdc_real;
    Ppv_in = Ipv_in*Vpv;
    Delta_PV = 0.5;
    Ppv_wanted = Ppv_in;
    
    if Control_pv == 2 % Cascade control
        if mod(Time,2e-4) == 0
            if Ppv_in < Ppv_pre
                Ppv_wanted  = Ppv_in - Delta_PV;
            end
            if Ppv_in > Ppv_pre
                Ppv_wanted  = Ppv_in + Delta_PV;
            end
        end
        if Ppv_out < 0
            Ppv_wanted = 180;
        end
        
        Ipv = Ppv_wanted/Vpv;
    else
        Ipv = 0;
    end
    
    % Converter wanter output voltage
    Vpv_conv = Vdc_command;
    
    
    % PV converter operates ?
    IO_pv_conv = IO_pv_conv_value;
    
    
    % Set the values for the next loop
    Ppv_pre = Ppv_in;
    Ppv_w_pre = Ppv_wanted;
    
    
    
    
    %% FC - control
    % FC converter operates ?
    IO_fc_conv = IO_fc_conv_value;
    
    %% D-ECMS:
%     Degradation-Conscious Equivalent Consumption Minimization Strategy for a Fuel Cell Hybrid System
    Pbatt_min=-150; Pbatt_max=800;
    SOC_min=60; SOC_max=90;
    Pfc_min=400;Pfc_max=1100;
    
    %define Matrix Aeq
    Aeq=[0 1 0;1 0 1];
    
    %define Matrix beq
    mu=0.6;
    beq=[1-2*mu*((SOC-0.5*(SOC_max+SOC_min))/(SOC_max+SOC_min)); Pload-Ppv_out];
    
    %define boundary conditions
    lb=[Pfc_min, 0, Pbatt_min];
    ub=[Pfc_max, 100, Pbatt_max];
    
    %define initial conditions
    x0=[1000, 0.1, 500];
    
    options = optimoptions('fmincon','Algorithm','sqp',...
        'Display','off','MaxFunctionEvaluations',500,'MaxIterations',100);
    [y,fval] = fmincon(@(x)decms(x,Vfc,Ifc_in,Ibatt_in,SOC),x0,[],[],Aeq,beq,lb,ub,[],options);
    
    Pfc=y(1); Pbatt=y(3); alpha=y(2);
    
    
    % Ifc command
    Ifc = Pfc/Vfc;
    
    % Converter wanted output voltage
    Vfc_conv = Vdc_command;
    if Ifc_in < Ifc
        Vfc_conv = 100;
    end
    
    
function f = decms(x,Vfc,Ifc_in,Ibatt_in,SOC)
    DT=200e-3;
    do = 0.5e-4;
    alpha = 4;
    FCcost = 525;
    Hcost = 2;
    BATcost = 640;
    Pfc_nom = 1000;
    Q = 15;
    dfc = (do/3600)*(1+alpha/(Pfc_nom^2)*(Vfc*Ifc_in-Pfc_nom)^2);
    dbat = (1/Q)*abs(weight_func_1(SOC)*weight_func_2(Ibatt_in)*Ibatt_in);
    mfc_deg = dfc * FCcost / Hcost;
    mbat_deg = dbat * BATcost / Hcost;
    f = (x(1)+x(2)*x(3)+ mfc_deg + mbat_deg)*DT;
    
function out = weight_func_1(SOC)
    out = 1+3.25*(1-SOC)^2;
    
function out = weight_func_2(Ibatt)
    Ibatt_nom = 2;
    if Ibatt >= 0
        out = 1+0.45*Ibatt/Ibatt_nom;
    else
        out = 1+0.55*abs(Ibatt)/Ibatt_nom;
    end

== matlab function simplified_powertrain/PEMFC matfunc V2/MATLAB Function ==
  settings: updateMethod=DISCRETE  sampleTime=1e-4
  data: U_H2 output; U_O2 output; R_ohm output; Ifc input; E_Ner output; E_ohm output; E_con output; E_act_steady output; E_act input; E_act_d output; limit output
function [U_H2,U_O2,R_ohm,E_Ner,E_ohm,E_con,E_act_steady,E_act_d,limit] = fcn(Ifc,E_act)
%     https://link.springer.com/article/10.1007/s40565-016-0196-5
%     Modeling and Simulation of a Proton Exchange Membrane Fuel Cell Alongside a Waste Heat Recovery System Based on the Organic Rankine Cycle in MATLAB/SIMULINK Environment
%     MATHEMATICAL MODELLING FOR PROTON EXCHANGE MEMBRANE FUEL CELL (PEMFC) 
%     https://www.scirp.org/pdf/epe_2020112310053180.pdf#page=17&zoom=100,72,604
%     H-Series Fuel Cell Stacks

    %% constants:
    R = 8.3145;
    Pstd = 101325;
    nF = 2*96485;
    C_act = 2;
    A = 19.6*4.0;
    T = 303.15;
    Nfc = 50;
    lambda = 14;
    l = 21e-4 * 10^-2;
%     l = 1.27e-4;
    
    J = Ifc/A;
    JM = 45/A;
    Pa = 1.45;
    Pc = 1;
    Tc = T-273.15;
    coeff = 1;
        
%     if Ifc <=0
%         Ifc = 40;
%     end
    
    PH2Osat = 10^(-2.18+2.95e-2*Tc-9.18e-5*Tc^2+1.44e-7*Tc^3);
    
    P_H2 = 0.5*PH2Osat*(exp(-(1.635*J/T^1.334))*(Pa/PH2Osat)-1);
    P_O2 = PH2Osat*(exp(-(4.192*J/T^1.334))*(Pc/PH2Osat)-1);
    

    %% Saturation at start
    if -1.87e-4*log(Ifc) > 0
        k = 0;
    else
        if -1.87e-4*log(Ifc) < -1.2
            k = -1.2;
        else
            k = -1.87e-4*log(Ifc);
        end
    end
    %% Nernst Voltage
    E_Ner = 1.229 + (T-298.15) * (-0.85e-3) + T*R/nF * log(P_H2*P_O2^0.5);
    
    %% Activation loss
    % Pressure not in Pa ?
    CO2 = (P_O2/(5.08e6))*exp(498/T);
    CH2 = (P_H2/(1.09e6))*exp(-77/T);
    E_act_steady=-0.9514 + T * (2.86e-3+2e-4*log(200)+4.3e-5*log(CH2)+7.4e-5*log(CO2)+k);
%     E_act_steady = -0.9514 + 3.12e-3*T + 7.4e-5*T*log(CO2) -1.87e-4*T*log(Ifc);
    
    %% Ohmic loss
    E_ohm = - Ifc*(l/((lambda*5.139e-3-3.26e-3)*exp(1268*(1/303-1/T))));
    R_ohm = (l/((lambda*5.139e-3-3.26e-3)*exp(1268*(1/303-1/T))));
    
    %% Concentration loss
%     if T>= 312.15
%         E_con = (1.1e-4-1.2e-6*(T-273.15))*exp(8*Ifc/40);
%     else
%         E_con = (3.3e-3-8.2e-5*(T-273.15))*exp(8*Ifc/40);
%     end

%     E_con = 3*R*T/(2*nF)*log(1-J/JM)-1.5607*R*T/(2*nF);
        if J/JM < 1
        E_con = 3*R*T/(2*nF)*log(1-J/JM)-1.5607*R*T/(2*nF);
    else
%         E_con = -abs(3*R*T/(2*nF)*log(complex(1-J/(JM-0.001)))-1.5607*R*T/(2*nF));
        E_con = 3*R*T/(2*nF)*log(J/JM)-1.5607*R*T/(2*nF);
    end
    
    %% with coefficient
    E_con = coeff * E_con;
    E_act_steady = coeff * E_act_steady;
    E_ohm = coeff * E_ohm;
    E_Ner = coeff * E_Ner;
    
        
    %% activation dynamic loss:
    below = -E_act_steady-E_con;
    E_act_d = (Ifc/C_act)*(1-E_act/below);
%     E_act_d = 0;

    %% Fuel utilization
    U_H2 = 60000*Ifc*R*T*Nfc/(nF*1.16*1*0.9995*Pstd);
    
    %% Air utilization
    U_O2 = 60000*Ifc*R*T*Nfc/(2*nF*0.0181*1*0.21*Pstd);
    limit = 1;
    if J/JM >= 1
            E_con = 0;
            E_act_steady = 0;
            E_ohm = 0;
            E_act_d = 0;
            E_Ner = -35*Ifc;
            if E_Ner <= 0
                E_Ner = 0;
            end
            limit = 0;
    end
end
